simulink model "crane_model"  (R2020b)
settings: Solver=ode1  StartTime=0.0  StopTime=60  FixedStep=0.01  RelTol=1e-3  EnableMultiTasking=on
Description:
  | Real-Time Van der Pol Simulation
  | 
  | This demonstration shows a real-time version of the Simulink Van der Pol
  | simulation demo. This model does not need any external signals, so it does
  | not need any data acquisition hardware or driver. This makes the model ideal
  | for first experiments with Real-Time Windows Target, without need to
  | worry about proper I/O hardware configuration.
  | 
  | How to run this demo:
  | 
  |   1. Build the model using Tools -> Real-Time Workshop -> Build Model.
  |   2. Connect to the real-time code using Simulation -> Connect to target.
  |   3. Start the real-time execution using Simulation -> Start real-time code.
settings Model: SimulationMode=external  Creator=Houska  LastModifiedBy=Admin
settings DataIOCC: LimitDataPoints=on  SaveFormat=Array  SignalLoggingSaveFormat=ModelDataLogs  SaveOutput=off  SaveTime=off  ReturnWorkspaceOutputs=off  SignalLoggingName=logsOut
settings OptimizationCC: ExpressionDepthLimit=2147483647  InitFltsAndDblsToZero=on  LifeSpan=inf
settings DebuggingCC: SaveWithParameterizedLinksMsg=none  UnderspecifiedInitializationDetection=Classic  MergeDetectMultiDrivingBlocksExec=none  SignalResolutionControl=TryResolveAllWithWarning  MultiTaskDSMMsg=warning  MultiTaskCondExecSysMsg=none  FcnCallInpInsideContextMsg=warning  StateNameClashWarn=warning  SFUnexpectedBacktrackingDiag=warning  SFNoUnconditionalDefaultTransitionDiag=warning  SFExecutionAtInitializationDiag=none  ArithmeticOperatorsInVariantConditions=warning
settings HardwareCC: ProdBitPerPointer=32  ProdBitPerSizeT=32  ProdBitPerPtrDiffT=32  ProdLargestAtomicFloat=None  ProdWordSize=32  ProdHWDeviceType=32-bit Real-Time Windows Target  TargetHWDeviceType=32-bit Generic  ProdEqTarget=off
settings ModelReferenceCC: PropagateSignalLabelsOutOfModel=off
settings SFSimCC: SimUseLocalCustomCode=off  CustomCodeUndefinedFunction=UseInterfaceOnly
settings RTWCC: Description=crane3d (Visual C/C++)  SystemTargetFile=rtcon_crane3d_USB2.tlc  TemplateMakefile=crane3d_vc_USB2_x64.tmf  RTWUseLocalCustomCode=off
settings CodeAppCC: StateflowObjectComments=on
settings STFCustomTargetCC: ModelReferenceCompliant=off  ConcurrentExecutionCompliant=off  CombineOutputUpdateFcns=on  MatFileLogging=on  GRTInterface=off  SystemTargetFile=rtcon_crane3d_USB2.tlc
settings GRTTargetCC: TargetLangStandard=C89/C90 (ANSI)  ModelReferenceCompliant=off  ParMdlRefBuildCompliant=off  CompOptLevelCompliant=off  ConcurrentExecutionCompliant=off  UseToolchainInfoCompliant=off  ExtMode=on  ExtModeMexFile=rtcon_ext_comm
settings ConfigComp: CovMetricSettings=dw  CovSaveCumulativeToWorkspaceVar=on  CovSaveSingleToWorkspaceVar=on  CovExternalEMLEnable=off  CovSFcnEnable=off

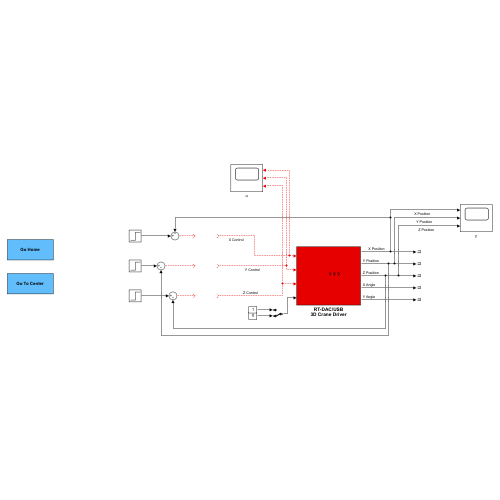
[thumbnail: Simulink's stored preview of the top-level diagram]
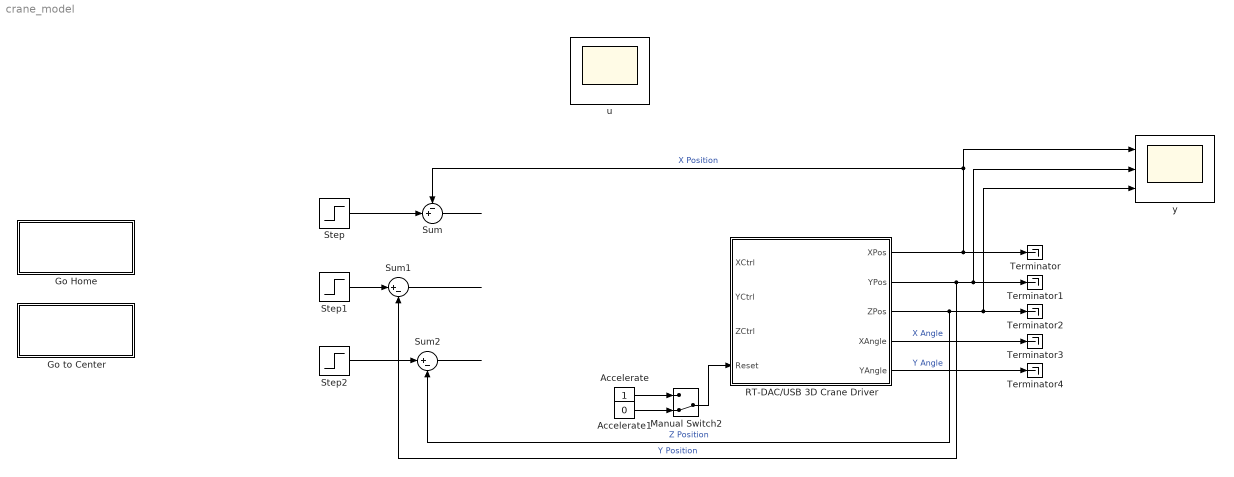
== system crane_model ==
  Accelerate : Constant
  Accelerate1 : Constant  Value=0
  Go Home : Subsystem
      settings: OpenFcn=BasicTestFunction( 'GoHomeXYZ', 0.5, 'Go Home !!!' );
      mask Display: fprintf( 'Go Home' )
  Go to Center : Subsystem
      settings: OpenFcn=BasicTestFunction( 'GotoCenter', 0.5, 'Go To Center !!!', 0 );
      mask Display: fprintf( 'Go To Center' )
  Manual Switch2 : ManualSwitch  CurrentSetting=0
  RT-DAC/USB 3D Crane Driver : Subsystem
      mask Display: image(imread('crane.jpeg'))
  Step : Step  Time=0  After=0.6  SampleTime=0
  Step1 : Step  Time=0  After=0.6  SampleTime=0
  Step2 : Step  Time=0  After=0.6  SampleTime=0
  Sum : Sum  Inputs=-+|
  Sum1 : Sum  Inputs=|+-
  Sum2 : Sum  Inputs=|+-
  Terminator{,1..4} (5 alike) : Terminator
  u : Scope  NumInputPorts=3
  y : Scope  NumInputPorts=3
  wires:
  RT-DAC/USB 3D Crane Driver/1(XPos) -> y/1, Sum/1, Terminator/1  "X Position"
  RT-DAC/USB 3D Crane Driver/2(YPos) -> Sum1/2, y/2, Terminator1/1  "Y Position"
  RT-DAC/USB 3D Crane Driver/3(ZPos) -> Sum2/2, y/3, Terminator2/1  "Z Position"
  ? -> u/3, RT-DAC/USB 3D Crane Driver/3(ZCtrl)  "Z Control"
  ? -> RT-DAC/USB 3D Crane Driver/2(YCtrl), u/2  "Y Control"
  RT-DAC/USB 3D Crane Driver/4(XAngle) -> Terminator3/1  "X Angle"
  RT-DAC/USB 3D Crane Driver/5(YAngle) -> Terminator4/1  "Y Angle"
  Accelerate1/1 -> Manual Switch2/2
  Manual Switch2/1 -> RT-DAC/USB 3D Crane Driver/4(Reset)
  Accelerate/1 -> Manual Switch2/1
  Sum/1 -> ?
  Step/1 -> Sum/2
  ? -> u/1, RT-DAC/USB 3D Crane Driver/1(XCtrl)  "X Control"
  Sum1/1 -> ?
  Sum2/1 -> ?
  Step1/1 -> Sum1/1
  Step2/1 -> Sum2/1

== system crane_model/Go Home ==

== system crane_model/Go to Center ==

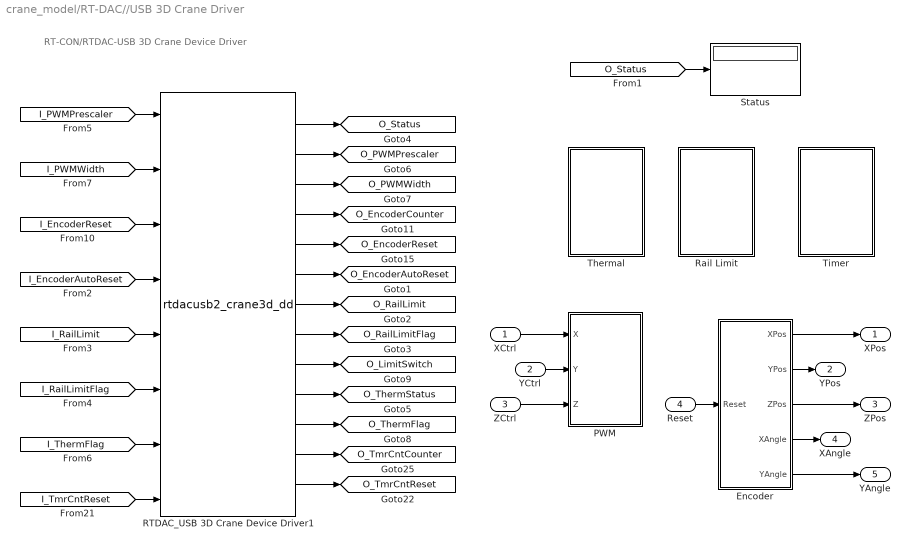
== system crane_model/RT-DAC//USB 3D Crane Driver ==
  note: RT-CON/RTDAC-USB 3D Crane Device Driver
  XCtrl : Inport
  YCtrl : Inport  Port=2
  ZCtrl : Inport  Port=3
  Reset : Inport  Port=4
  Encoder : Subsystem
  PWM : Subsystem
      mask Display: disp('PWM')
  RTDAC_USB 3D Crane Device Driver1 : S-Function  FunctionName=rtdacusb2_crane3d_dd  Parameters=-1, 0.01  SFunctionDeploymentMode=off  EnableBusSupport=off
  Rail Limit : Subsystem
      mask Display: disp('Rail\nLimit')
  Status : Display
  Thermal : Subsystem
      mask Display: disp('Thermal')
  Timer : Subsystem
      mask Display: disp('Timer')
  XPos : Outport  VectorParamsAs1DForOutWhenUnconnected=off
  YPos : Outport  Port=2  VectorParamsAs1DForOutWhenUnconnected=off
  ZPos : Outport  Port=3  VectorParamsAs1DForOutWhenUnconnected=off
  XAngle : Outport  Port=4  VectorParamsAs1DForOutWhenUnconnected=off
  YAngle : Outport  Port=5  VectorParamsAs1DForOutWhenUnconnected=off
  tag scope: O_EncoderAutoReset=global, O_EncoderCounter=global, O_EncoderReset=global, O_LimitSwitch=global, O_PWMPrescaler=global, O_PWMWidth=global, O_RailLimit=global, O_RailLimitFlag=global, O_Status=global, O_ThermFlag=global, O_ThermStatus=global, O_TmrCntCounter=global, O_TmrCntReset=global
  wires:
  [O_Status] -> Status/1
  XCtrl/1 -> PWM/1(X)
  YCtrl/1 -> PWM/2(Y)
  Reset/1 -> Encoder/1(Reset)
  Encoder/1(XPos) -> XPos/1
  Encoder/2(YPos) -> YPos/1
  Encoder/3(ZPos) -> ZPos/1
  RTDAC_USB 3D Crane Device Driver1/1 -> [O_Status]
  [I_PWMPrescaler] -> RTDAC_USB 3D Crane Device Driver1/1
  [I_PWMWidth] -> RTDAC_USB 3D Crane Device Driver1/2
  ZCtrl/1 -> PWM/3(Z)
  RTDAC_USB 3D Crane Device Driver1/2 -> [O_PWMPrescaler]
  RTDAC_USB 3D Crane Device Driver1/3 -> [O_PWMWidth]
  [I_TmrCntReset] -> RTDAC_USB 3D Crane Device Driver1/8
  RTDAC_USB 3D Crane Device Driver1/12 -> [O_TmrCntCounter]
  RTDAC_USB 3D Crane Device Driver1/13 -> [O_TmrCntReset]
  [I_EncoderReset] -> RTDAC_USB 3D Crane Device Driver1/3
  RTDAC_USB 3D Crane Device Driver1/4 -> [O_EncoderCounter]
  RTDAC_USB 3D Crane Device Driver1/5 -> [O_EncoderReset]
  Encoder/4(XAngle) -> XAngle/1
  Encoder/5(YAngle) -> YAngle/1
  [I_EncoderAutoReset] -> RTDAC_USB 3D Crane Device Driver1/4
  RTDAC_USB 3D Crane Device Driver1/6 -> [O_EncoderAutoReset]
  [I_RailLimit] -> RTDAC_USB 3D Crane Device Driver1/5
  [I_RailLimitFlag] -> RTDAC_USB 3D Crane Device Driver1/6
  [I_ThermFlag] -> RTDAC_USB 3D Crane Device Driver1/7
  RTDAC_USB 3D Crane Device Driver1/8 -> [O_RailLimitFlag]
  RTDAC_USB 3D Crane Device Driver1/7 -> [O_RailLimit]
  RTDAC_USB 3D Crane Device Driver1/10 -> [O_ThermStatus]
  RTDAC_USB 3D Crane Device Driver1/11 -> [O_ThermFlag]
  RTDAC_USB 3D Crane Device Driver1/9 -> [O_LimitSwitch]

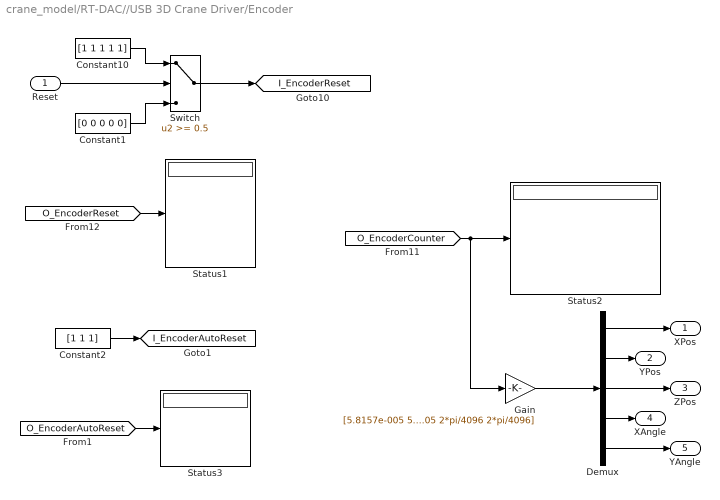
== system crane_model/RT-DAC//USB 3D Crane Driver/Encoder ==
  Reset : Inport
  Constant1 : Constant  Value=[0 0 0 0 0]
  Constant10 : Constant  Value=[1 1 1 1 1]
  Constant2 : Constant  Value=[1 1 1]
  Demux : Demux  Outputs=5
  Gain : Gain  Gain=[5.8157e-005 5.8157e-005 2.2150e-005 2*pi/4096 2*pi/4096]  SaturateOnIntegerOverflow=on  OutDataTypeStr=Inherit: Same as input  ParamDataTypeStr=Inherit: Same as input
  Status1 : Display
  Status2 : Display
  Status3 : Display
  Switch : Switch  Threshold=0.5  InputSameDT=on
  XPos : Outport  VectorParamsAs1DForOutWhenUnconnected=off
  YPos : Outport  Port=2  VectorParamsAs1DForOutWhenUnconnected=off
  ZPos : Outport  Port=3  VectorParamsAs1DForOutWhenUnconnected=off
  XAngle : Outport  Port=4  VectorParamsAs1DForOutWhenUnconnected=off
  YAngle : Outport  Port=5  VectorParamsAs1DForOutWhenUnconnected=off
  tag scope: I_EncoderAutoReset=global, I_EncoderReset=global
  wires:
  [O_EncoderReset] -> Status1/1
  [O_EncoderCounter] -> Status2/1, Gain/1
  Demux/1 -> XPos/1
  Demux/2 -> YPos/1
  Demux/3 -> ZPos/1
  Reset/1 -> Switch/2
  Switch/1 -> [I_EncoderReset]
  Constant10/1 -> Switch/1
  Constant1/1 -> Switch/3
  Gain/1 -> Demux/1
  Demux/4 -> XAngle/1
  Demux/5 -> YAngle/1
  Constant2/1 -> [I_EncoderAutoReset]
  [O_EncoderAutoReset] -> Status3/1

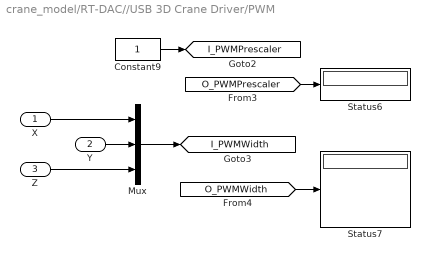
== system crane_model/RT-DAC//USB 3D Crane Driver/PWM ==
  X : Inport
  Y : Inport  Port=2
  Z : Inport  Port=3
  Constant9 : Constant
  Mux : Mux  Inputs=3
  Status6 : Display
  Status7 : Display
  tag scope: I_PWMPrescaler=global, I_PWMWidth=global
  wires:
  [O_PWMWidth] -> Status7/1
  [O_PWMPrescaler] -> Status6/1
  Constant9/1 -> [I_PWMPrescaler]
  X/1 -> Mux/1
  Y/1 -> Mux/2
  Mux/1 -> [I_PWMWidth]
  Z/1 -> Mux/3

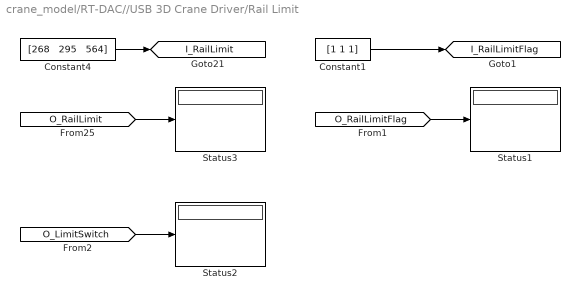
== system crane_model/RT-DAC//USB 3D Crane Driver/Rail Limit ==
  Constant1 : Constant  Value=[1 1 1]
  Constant4 : Constant  Value="[268   295   564]"
  Status1 : Display
  Status2 : Display
  Status3 : Display
  tag scope: I_RailLimit=global, I_RailLimitFlag=global
  wires:
  [O_RailLimit] -> Status3/1
  Constant4/1 -> [I_RailLimit]
  [O_RailLimitFlag] -> Status1/1
  Constant1/1 -> [I_RailLimitFlag]
  [O_LimitSwitch] -> Status2/1

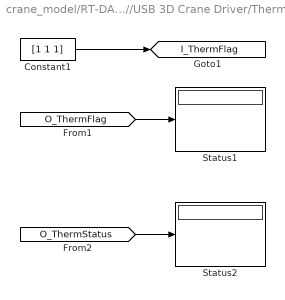
== system crane_model/RT-DAC//USB 3D Crane Driver/Thermal ==
  Constant1 : Constant  Value=[1 1 1]
  Status1 : Display
  Status2 : Display
  tag scope: I_ThermFlag=global
  wires:
  [O_ThermStatus] -> Status2/1
  Constant1/1 -> [I_ThermFlag]
  [O_ThermFlag] -> Status1/1

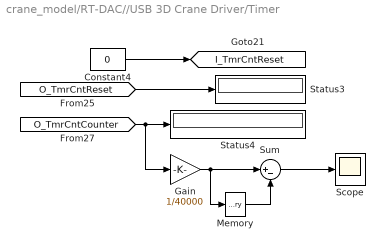
== system crane_model/RT-DAC//USB 3D Crane Driver/Timer ==
  Constant4 : Constant  Value=0
  Gain : Gain  Gain=1/40000  SaturateOnIntegerOverflow=on  OutDataTypeStr=Inherit: Same as input  ParamDataTypeStr=Inherit: Same as input
  Memory : Memory
  Scope : Scope
  Status3 : Display
  Status4 : Display
  Sum : Sum  Inputs=|+-  InputSameDT=on  SaturateOnIntegerOverflow=on  OutDataTypeStr=Inherit: Same as first input
  tag scope: I_TmrCntReset=global
  wires:
  Constant4/1 -> [I_TmrCntReset]
  [O_TmrCntReset] -> Status3/1
  [O_TmrCntCounter] -> Status4/1, Gain/1
  Gain/1 -> Sum/1, Memory/1
  Memory/1 -> Sum/2
  Sum/1 -> Scope/1
